simulink model "test_PP_full_state"  (R2019b)
settings: Solver=FixedStepAuto  StartTime=0.0  StopTime=20.0  FixedStep=1e-4  RelTol=1e-3
values from neighbouring files (symbols this model uses):
  A_sys = double(subs(A_pi, Params, Params_value))    [Sys_Linearization.m]
  B_sys = double(subs(B_pi, Params, Params_value))    [Sys_Linearization.m]
settings Model: Creator=francescoceresetti  LastModifiedBy=francescoceresetti

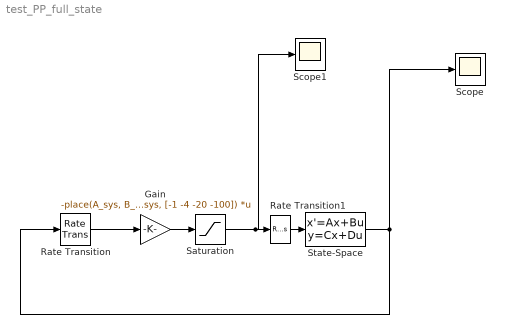
== system test_PP_full_state ==
  Gain : Gain  Gain=-place(A_sys, B_sys, [-1 -4 -20 -100])  Multiplication=Matrix(K*u)
  Rate Transition : RateTransition  OutPortSampleTime=2e-3
  Rate Transition1 : RateTransition  OutPortSampleTime=1e-4
  Saturation : Saturate  UpperLimit=22e-3  LowerLimit=-22e-3
  Scope : Scope
  Scope1 : Scope
  State-Space : StateSpace  A=A_sys  B=B_sys  C=eye(4)  D=zeros(4,1)  InitialCondition=[0 0 0.1 0]
  wires:
  Gain/1 -> Saturation/1
  Saturation/1 -> Scope1/1, Rate Transition1/1
  Rate Transition/1 -> Gain/1
  State-Space/1 -> Rate Transition/1, Scope/1
  Rate Transition1/1 -> State-Space/1
